simulink model "C172S_YawDamper_V2_Actuator"  (R2026a)
settings: Solver=ode4  StartTime=0  StopTime=30  FixedStep=0.01
InitFcn:
  | yd2Data = c172sLateralDirectionalData();
  | [~,yd2Plant] = c172sLateralDirectionalPlant(yd2Data);
  | yd2Controller = c172sYawDamperData();
  | yd2Actuator = c172sRudderActuatorData();
  | if ~strcmp(yd2Data.model.version,yd2Actuator.requiredPlantVersion), error('Yaw Damper V2 plant dependency mismatch.'); end
  | if ~strcmp(yd2Controller.artifactRevision,yd2Actuator.requiredYawDamperRevision), error('Yaw Damper V2 controller dependency mismatch.'); end
  | if ~strcmp(yd2Actuator.artifactRevision,'YD-V2-AUDIT-MATLAB-R1'), error('Yaw Damper V2 audit revision mismatch.'); end
  | A_yd2 = yd2Plant.A; B_yd2 = yd2Plant.B;
  | C_yd2 = yd2Plant.C; D_yd2 = yd2Plant.D;
  | Kr_yd2 = yd2Controller.rudderGain_s;
  | Tw_yd2 = yd2Controller.washoutTimeConstant_s;
  | Ts_yd2 = yd2Actuator.sensor.filterTimeConstant_s;
  | tauActuator_yd2 = yd2Actuator.dynamics.timeConstant_s;
  | delaySampleTime_yd2 = yd2Actuator.sensor.nominalDelay_s;
  | autoRudderLower_yd2_rad = yd2Actuator.authority.lowerLimit_rad;
  | autoRudderUpper_yd2_rad = yd2Actuator.authority.upperLimit_rad;
  | rateLower_yd2_radps = -deg2rad(yd2Actuator.dynamics.rateLimit_degps);
  | rateUpper_yd2_radps = deg2rad(yd2Actuator.dynamics.rateLimit_degps);
  | totalRudderLower_yd2_rad = yd2Actuator.physicalTravel.lowerLimit_rad;
  | totalRudderUpper_yd2_rad = yd2Actuator.physicalTravel.upperLimit_rad;
  | if ~exist('deltaACommand_yd2_rad','var'), deltaACommand_yd2_rad = deg2rad(1.0); end
  | if ~exist('deltaRCommand_yd2_rad','var'), deltaRCommand_yd2_rad = deg2rad(1.0); end
  | if ~exist('noiseAmplitude_yd2_radps','var'), noiseAmplitude_yd2_radps = 0.0; end
  | if ~exist('noiseFrequency_yd2_radps','var'), noiseFrequency_yd2_radps = 50.0; end
  | if ~exist('x0_yd2','var'), x0_yd2 = zeros(5,1); end
  | if ~exist('rDelay0_yd2_radps','var'), rDelay0_yd2_radps = x0_yd2(3); end
  | if ~exist('rSensor0_yd2_radps','var'), rSensor0_yd2_radps = 0.0; end
  | if ~exist('xw0_yd2_radps','var'), xw0_yd2_radps = 0.0; end
  | if ~exist('deltaRAuto0_yd2_rad','var'), deltaRAuto0_yd2_rad = 0.0; end
undefined symbols (not defined in the file or in its folder): deltaACommand_yd2_rad, deltaRAuto0_yd2_rad, deltaRCommand_yd2_rad, noiseAmplitude_yd2_radps, noiseFrequency_yd2_radps, rDelay0_yd2_radps, rSensor0_yd2_radps, x0_yd2, xw0_yd2_radps
settings Model: Creator=Shahi  LastModifiedBy=Shahi

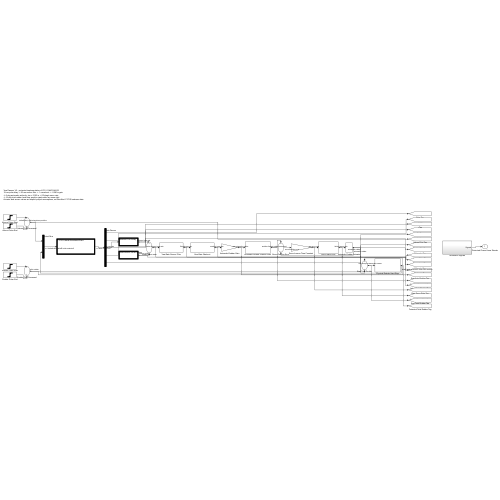
[thumbnail: Simulink's stored preview of the top-level diagram]
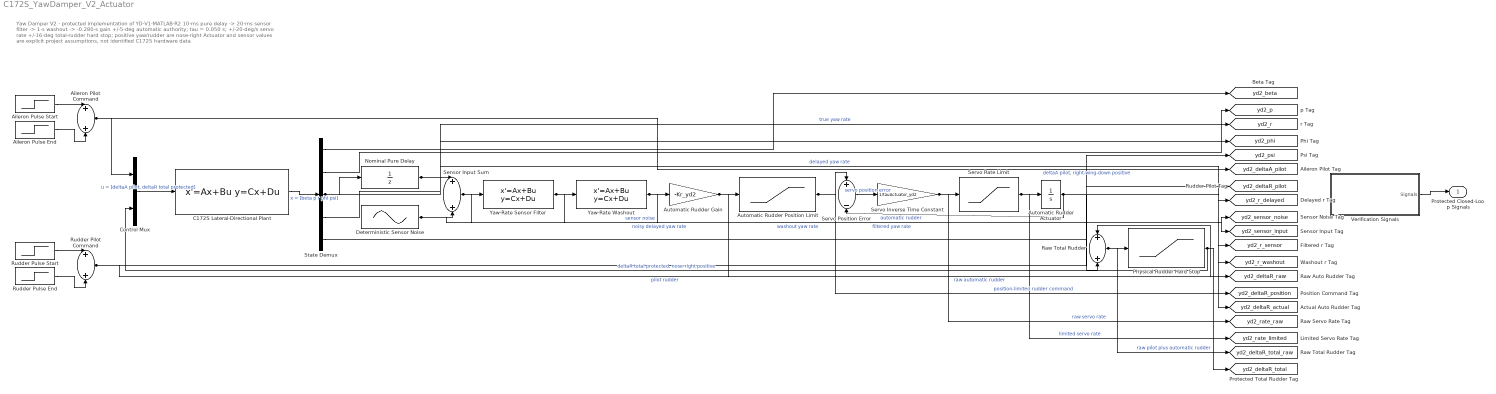
== system C172S_YawDamper_V2_Actuator ==
  note: Yaw Damper V2 - protected implementation of YD-V1-MATLAB-R2
      | 10-ms pure delay -> 20-ms sensor filter -> 1-s washout -> -0.280-s gain
      | +/-5-deg automatic authority; tau = 0.050 s; +/-20-deg/s servo rate
      | +/-16-deg total-rudder hard stop; positive yaw/rudder are nose-right
      | Actuator and sensor values are explicit project assumptions, not identified C172S hardware data
  Aileron Pilot Command : Sum
  Aileron Pulse End : Step  FinalValue=-deltaACommand_yd2_rad  SampleTime=0
  Aileron Pulse Start : Step  Time=0  FinalValue=deltaACommand_yd2_rad  SampleTime=0
  Automatic Rudder Actuator : Integrator  InitialCondition=deltaRAuto0_yd2_rad
  Automatic Rudder Gain : Gain  Gain=-Kr_yd2
  Automatic Rudder Position Limit : Saturate  UpperLimit=autoRudderUpper_yd2_rad  LowerLimit=autoRudderLower_yd2_rad
  C172S Lateral-Directional Plant : StateSpace  A=A_yd2  B=B_yd2  C=C_yd2  D=D_yd2  InitialCondition=x0_yd2
  Control Mux : Mux  Inputs=2
  Deterministic Sensor Noise : Sin  Amplitude=noiseAmplitude_yd2_radps  Frequency=noiseFrequency_yd2_radps  SampleTime=0
  Nominal Pure Delay : UnitDelay  InitialCondition=rDelay0_yd2_radps  SampleTime=delaySampleTime_yd2
  Physical Rudder Hard Stop : Saturate  UpperLimit=totalRudderUpper_yd2_rad  LowerLimit=totalRudderLower_yd2_rad
  Raw Total Rudder : Sum
  Rudder Pilot Command : Sum
  Rudder Pulse End : Step  Time=6  FinalValue=-deltaRCommand_yd2_rad  SampleTime=0
  Rudder Pulse Start : Step  Time=5  FinalValue=deltaRCommand_yd2_rad  SampleTime=0
  Sensor Input Sum : Sum
  Servo Inverse Time Constant : Gain  Gain=1/tauActuator_yd2
  Servo Position Error : Sum  Inputs=+-
  Servo Rate Limit : Saturate  UpperLimit=rateUpper_yd2_radps  LowerLimit=rateLower_yd2_radps
  State Demux : Demux  Outputs=5
  Verification Signals : Subsystem
  Yaw-Rate Sensor Filter : StateSpace  A=-1/Ts_yd2  B=1/Ts_yd2  D=0  InitialCondition=rSensor0_yd2_radps
  Yaw-Rate Washout : StateSpace  A=-1/Tw_yd2  B=1/Tw_yd2  C=-1  InitialCondition=xw0_yd2_radps
  Protected Closed-Loop Signals : Outport
  tag scope: yd2_beta=global, yd2_deltaA_pilot=global, yd2_deltaR_actual=global, yd2_deltaR_pilot=global, yd2_deltaR_position=global, yd2_deltaR_raw=global, yd2_deltaR_total=global, yd2_deltaR_total_raw=global, yd2_p=global, yd2_phi=global, yd2_psi=global, yd2_r=global, yd2_r_delayed=global, yd2_r_sensor=global, yd2_r_washout=global, yd2_rate_limited=global, yd2_rate_raw=global, yd2_sensor_input=global, yd2_sensor_noise=global
  wires:
  Aileron Pulse Start/1 -> Aileron Pilot Command/1
  Aileron Pulse End/1 -> Aileron Pilot Command/2
  Rudder Pulse Start/1 -> Rudder Pilot Command/1
  Rudder Pulse End/1 -> Rudder Pilot Command/2
  Aileron Pilot Command/1 -> Control Mux/1, [yd2_deltaA_pilot]  "deltaA pilot, right-wing-down positive"
  Physical Rudder Hard Stop/1 -> Control Mux/2, [yd2_deltaR_total]  "deltaR total protected, nose-right positive"
  Control Mux/1 -> C172S Lateral-Directional Plant/1  "u = [deltaA pilot, deltaR total protected]"
  C172S Lateral-Directional Plant/1 -> State Demux/1  "x = [beta p r phi psi]"
  State Demux/3 -> Nominal Pure Delay/1, [yd2_r]  "true yaw rate"
  Nominal Pure Delay/1 -> Sensor Input Sum/1, [yd2_r_delayed]  "delayed yaw rate"
  Deterministic Sensor Noise/1 -> Sensor Input Sum/2, [yd2_sensor_noise]  "sensor noise"
  Sensor Input Sum/1 -> Yaw-Rate Sensor Filter/1, [yd2_sensor_input]  "noisy delayed yaw rate"
  Yaw-Rate Sensor Filter/1 -> Yaw-Rate Washout/1, [yd2_r_sensor]  "filtered yaw rate"
  Yaw-Rate Washout/1 -> Automatic Rudder Gain/1, [yd2_r_washout]  "washout yaw rate"
  Automatic Rudder Gain/1 -> Automatic Rudder Position Limit/1, [yd2_deltaR_raw]  "raw automatic rudder"
  Automatic Rudder Position Limit/1 -> Servo Position Error/1, [yd2_deltaR_position]  "position-limited rudder command"
  Automatic Rudder Actuator/1 -> Servo Position Error/2, Raw Total Rudder/2, [yd2_deltaR_actual]  "automatic rudder"
  Servo Position Error/1 -> Servo Inverse Time Constant/1  "servo position error"
  Servo Inverse Time Constant/1 -> Servo Rate Limit/1, [yd2_rate_raw]  "raw servo rate"
  Servo Rate Limit/1 -> Automatic Rudder Actuator/1, [yd2_rate_limited]  "limited servo rate"
  Rudder Pilot Command/1 -> Raw Total Rudder/1, [yd2_deltaR_pilot]  "pilot rudder"
  Raw Total Rudder/1 -> Physical Rudder Hard Stop/1, [yd2_deltaR_total_raw]  "raw pilot plus automatic rudder"
  Verification Signals/1(Signals) -> Protected Closed-Loop Signals/1
  State Demux/1 -> [yd2_beta]
  State Demux/2 -> [yd2_p]
  State Demux/4 -> [yd2_phi]
  State Demux/5 -> [yd2_psi]

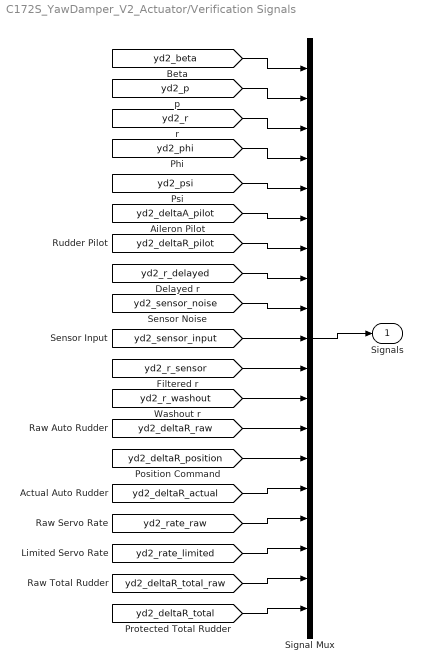
== system C172S_YawDamper_V2_Actuator/Verification Signals ==
  Signal Mux : Mux  Inputs=19
  Signals : Outport
  wires:
  [yd2_beta] -> Signal Mux/1
  [yd2_p] -> Signal Mux/2
  [yd2_r] -> Signal Mux/3
  [yd2_phi] -> Signal Mux/4
  [yd2_psi] -> Signal Mux/5
  [yd2_deltaA_pilot] -> Signal Mux/6
  [yd2_deltaR_pilot] -> Signal Mux/7
  [yd2_r_delayed] -> Signal Mux/8
  [yd2_sensor_noise] -> Signal Mux/9
  [yd2_sensor_input] -> Signal Mux/10
  [yd2_r_sensor] -> Signal Mux/11
  [yd2_r_washout] -> Signal Mux/12
  [yd2_deltaR_raw] -> Signal Mux/13
  [yd2_deltaR_position] -> Signal Mux/14
  [yd2_deltaR_actual] -> Signal Mux/15
  [yd2_rate_raw] -> Signal Mux/16
  [yd2_rate_limited] -> Signal Mux/17
  [yd2_deltaR_total_raw] -> Signal Mux/18
  [yd2_deltaR_total] -> Signal Mux/19
  Signal Mux/1 -> Signals/1
